simulink model "TV_lisb"  (R2024b)
settings: Solver=ode45  StartTime=0.0  StopTime=10  MaxStep=0.05  RelTol=1e-3
model workspace: external: MATLAB File C:\Users\USER\Documents\MATLAB\NR\TV_lisb_helper_file.m (data not in the file)
values from neighbouring files (symbols this model uses):
  b = 0.1    [TV_lisb_helper_file.m]
  C1 = 1.28    [TV_lisb_helper_file.m]
  C2 = 23.99    [TV_lisb_helper_file.m]
  C3 = 0.52    [TV_lisb_helper_file.m]
  C_d = 0.89    [TV_lisb_helper_file.m]
  C_roll = 0.01    [TV_lisb_helper_file.m]
  frontal_area = 1.35    [TV_lisb_helper_file.m]
  g = 9.8    [TV_lisb_helper_file.m]
  I_w = 1.5    [TV_lisb_helper_file.m]
  Izz = 3000    [TV_lisb_helper_file.m]
  lf = 1.5    [TV_lisb_helper_file.m]
  lr = 1.5    [TV_lisb_helper_file.m]
  M = 300    [TV_lisb_helper_file.m]
  rho = 1.223    [TV_lisb_helper_file.m]
  tr = 1    [TV_lisb_helper_file.m]
  wr = 0.22    [TV_lisb_helper_file.m]
libraries: simulink x1
(part 1 of 2)
settings Model: SnapshotBufferSize=100  SnapshotInterval=1  Creator=USER  LastModifiedBy=USER

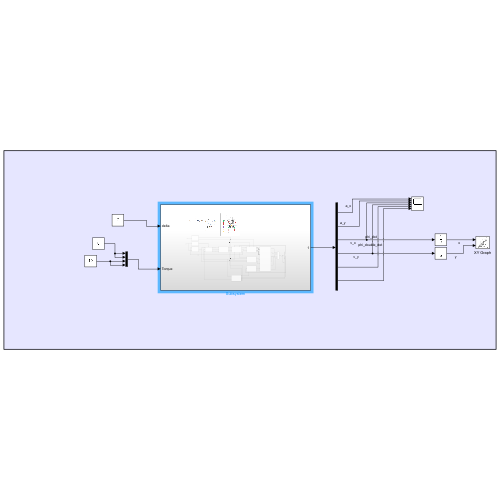
[thumbnail: Simulink's stored preview of the top-level diagram]
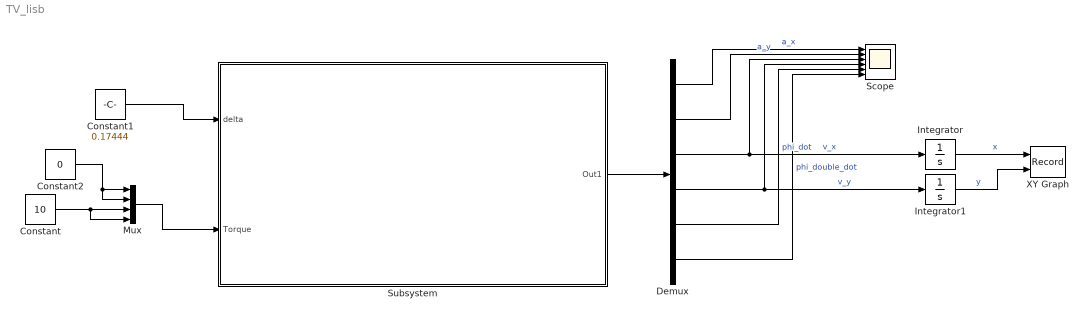
== system TV_lisb ==
  Constant : Constant  Value=10
  Constant1 : Constant  Value=0.17444
  Constant2 : Constant  Value=0
  Demux : Demux  Outputs=6
  Integrator : Integrator
  Integrator1 : Integrator
  Mux : Mux
  Scope : Scope  NumInputPorts=6
  Subsystem : Subsystem
  XY Graph : Record  FileSettingsInternal="{\"entries\":[{\"content\":{\"excelSettings\":{\"content\":{},\"type\":\"Streamout.ExcelSettings\"}},\"type\":\"Streamout.FileSettingStorage\",\"uuid\":\"\"}],\"packageUris\":[\"http:\\/\\/schema.mathworks.com\\/mf0\\/streamout_blocks\\/R2020a\"],\"version\":\"1.0\"}"  Layout=[1 1]  SignalsInternal="{\"entries\":[{\"content\":{\"signals\":[{\"content\":{\"blockPath\":[],\"dimensions\":[1],\"domain\":\"\",\"lineColor\":\"#a2142f\",\"plots\":[ 1 ],\"port\":1,\"sid\":[\"\"],\"signalID\":1,\"signalName\":\"x\"},\"type\":\"RecordBlkView.Signal\",\"uuid\":\"\"},{\"content\":{\"blockPath\":[],\"dimensions\":[1],\"domain\":\"\",\"lineColor\":\"#139fff\",\"plots\":[ 1 ],\"port\":2,\"sid\":[\"\"],\"signalID\":2,\"signalName\":\"y\"},\"type\":\"RecordBlkView.Signal\",\"uuid\":\"\"}]},\"type\":\"RecordBlkView.InputSignals\",\"uuid\":\"\"}],\"packageUris\":[\"http:\\/\\/schema.mathworks.com\\/mf0\\/streamout_blocks\\/R2020a\"],\"version\":\"1.0\"}"  VisualizationBindings="{\"xyplotplugin\":{\"info\":[{\"series\":[{\"bindingParametersList\":[{\"parameter\":\"X-Axis\",\"signalID\":1,\"signalName\":\"x\"},{\"parameter\":\"Y-Axis\",\"signalID\":2,\"signalName\":\"y\"}],\"seriesID\":0}],\"subplotID\":1}]}}"  CompatibilityTag=XY
  wires:
  Subsystem/1(Out1) -> Demux/1
  Demux/1 -> Scope/1  "a_x"
  Demux/2 -> Scope/2  "a_y"
  Demux/3 -> Scope/3, Integrator/1  "v_x"
  Demux/4 -> Scope/4, Integrator1/1  "v_y"
  Demux/5 -> Scope/5  "phi_dot"
  Demux/6 -> Scope/6  "phi_double_dot"
  Integrator/1 -> XY Graph/1  "x"
  Integrator1/1 -> XY Graph/2  "y"
  Constant1/1 -> Subsystem/1(delta)
  Mux/1 -> Subsystem/2(Torque)
  Constant/1 -> Mux/4, Mux/3
  Constant2/1 -> Mux/1, Mux/2

== system TV_lisb/Subsystem ==
  delta : Inport
  Torque : Inport  Port=2
  Accelerating_or_braking : Subsystem
  Aerodynamic Drag : Subsystem
  Demux : Demux  Outputs=6
  Mux : Mux  Inputs=6
      settings: DisplayOption=signals
  Rolling resistance : Subsystem
  Side Slip Angle : Subsystem
  Slip Ratios : Subsystem
      settings: PortSchema="{\"entries\":[{\"content\":{\"sides\":[{\"content\":{\"connectorIds\":[\"In1\",\"In2\",\"In3\"]},\"type\":\"ConnectorPlacement.EquallySpacedRectSide\",\"uuid\":\"f68f1183-9c60-479b-925c-3d4ffcaa1183\"},{\"content\":{\"connectorIds\":[\"Out1\",\"Out2\",\"Out3\"],\"side\":\"RIGHT\"},\"type\":\"ConnectorPlacement.EquallySpacedRectSide\",\"uuid\":\"3ccc78e5-55f6-4f64-bd15-35f9b9c5843d\"},{\"content\":{\"connectorIds\":[\"In4\"],\"side\":\"TOP\"},\"type\":\"ConnectorPlacement.EquallySpacedRectSide\",\"uuid\":\"873faff7-faeb-472b-bbf0-059c7e3a1cec\"}]},\"type\":\"ConnectorPlacement.EquallySpacedConnector\",\"uuid\":\"c1430164-14ee-465b-ad5a-b929bb7f1d2a\"}],\"packageUris\":[\"http://schema.mathworks.com/mf0/Connector/R2020b\"],\"version\":\"1.0\"}"
  Steering Kinematics : Subsystem
  Tire Model : Subsystem
  Torque and force equilibrium : Subsystem
  Unit Delay : UnitDelay  SampleTime=-1  HasFrameUpgradeWarning=on
  Unit Delay2 : UnitDelay  SampleTime=-1  HasFrameUpgradeWarning=on
  Vertical Loads : Subsystem
      settings: PortSchema="{\"entries\":[{\"content\":{\"sides\":[{\"content\":{\"connectorIds\":[\"In1\",\"In2\"]},\"type\":\"ConnectorPlacement.EquallySpacedRectSide\",\"uuid\":\"420474dd-77ae-41a3-b184-b8a376845dee\"},{\"content\":{\"connectorIds\":[\"Out1\",\"Out2\",\"Out3\"],\"side\":\"RIGHT\"},\"type\":\"ConnectorPlacement.EquallySpacedRectSide\",\"uuid\":\"e98bfd49-6816-4384-b726-feedfd108428\"},{\"content\":{\"connectorIds\":[\"In3\",\"In4\"],\"side\":\"TOP\"},\"type\":\"ConnectorPlacement.EquallySpacedRectSide\",\"uuid\":\"bc3c4692-54cb-49d4-bb5f-a504cda1efb8\"},{\"content\":{\"connectorIds\":[\"In5\",\"Out4\"],\"side\":\"BOTTOM\"},\"type\":\"ConnectorPlacement.EquallySpacedRectSide\",\"uuid\":\"ec39efe8-9589-4d25-8c83-c5c7b2f70cfd\"}]},\"type\":\"ConnectorPlacement.EquallySpacedConnector\",\"uuid\":\"6b01247e-c69a-46fe-b6d9-037bfd45934f\"}],\"packageUris\":[\"http://schema.mathworks.com/mf0/Connector/R2020b\"],\"version\":\"1.0\"}"
  Wheel Dynamics : Subsystem
  Wheel To Vehicle Co-ordinate System : Subsystem
      settings: PortSchema="{\"entries\":[{\"content\":{\"sides\":[{\"content\":{\"connectorIds\":[\"In1\",\"In2\"]},\"type\":\"ConnectorPlacement.EquallySpacedRectSide\",\"uuid\":\"1d639fc9-362c-4114-a9a5-2cccb0aa4f8f\"},{\"content\":{\"connectorIds\":[\"Out1\",\"Out2\"],\"side\":\"RIGHT\"},\"type\":\"ConnectorPlacement.EquallySpacedRectSide\",\"uuid\":\"af7b8bc1-4639-4e57-ae25-0425d451201b\"},{\"content\":{\"connectorIds\":[\"In3\",\"In4\"],\"side\":\"TOP\"},\"type\":\"ConnectorPlacement.EquallySpacedRectSide\",\"uuid\":\"e7928f69-bff2-45cc-8c36-948ca369821c\"}]},\"type\":\"ConnectorPlacement.EquallySpacedConnector\",\"uuid\":\"c77d5f9f-6196-466d-893b-8bb143925d68\"}],\"packageUris\":[\"http://schema.mathworks.com/mf0/Connector/R2020b\"],\"version\":\"1.0\"}"
  Out1 : Outport
  wires:
  Steering Kinematics/1(delta_left) -> Side Slip Angle/4(delta_l), Rolling resistance/2(delta_left), Wheel To Vehicle Co-ordinate System/4(delta_left)
  Vertical Loads/4(Total_z_force) -> Rolling resistance/1(Total_z_force)
  Steering Kinematics/2(delta_right) -> Side Slip Angle/5(delta_r), Rolling resistance/3(delta_right), Wheel To Vehicle Co-ordinate System/3(delta_right)
  Accelerating_or_braking/1(Binary state) -> Slip Ratios/4(Binary state)
  Torque and force equilibrium/4(v_y) -> Mux/4  "v_y"
  Side Slip Angle/1(alpha) -> Slip Ratios/2(Alpha), Vertical Loads/5(alpha)
  Slip Ratios/3(Slip_ratio_lateral) -> Tire Model/3(Slip_ratio_lateral)
  Wheel To Vehicle Co-ordinate System/2(Wheel_forces_y_wrt_body) -> Torque and force equilibrium/2(Wheel_forces_y_wrt_body)
  Rolling resistance/1(Rolling_force_x_body) -> Torque and force equilibrium/3(Rolling_force_x_body)
  Torque and force equilibrium/3(v_x) -> Mux/3  "v_x"
  Aerodynamic Drag/1(F_body_drag) -> Torque and force equilibrium/5(F_body_drag)
  Tire Model/1(mu_longitudinal) -> Vertical Loads/1(mu_longitudinal)
  Wheel To Vehicle Co-ordinate System/1(Wheel_forces_x_wrt_body) -> Torque and force equilibrium/1(Wheel_forces_x_wrt_body)
  Slip Ratios/1(Slip_ratio_resultant) -> Tire Model/1(Slip_ratio_resultant)
  Vertical Loads/3(Wheel_force_res) -> Unit Delay2/1
  Torque and force equilibrium/5(phi_dot) -> Mux/5  "phi_dot"
  Tire Model/2(mu_lateral) -> Vertical Loads/2(mu_lateral)
  Torque and force equilibrium/6(phi_double_dot) -> Mux/6  "phi_double_dot"
  Side Slip Angle/2(Wheel_velocity) -> Slip Ratios/3(Wheel velocity)
  Rolling resistance/2(Rolling_force_y_body) -> Torque and force equilibrium/4(Rolling_force_y_body)
  Slip Ratios/2(Slip_ratio_longitudinal) -> Tire Model/2(Slip_ratio_longitudinal)
  Vertical Loads/2(Wheel_force_y) -> Wheel To Vehicle Co-ordinate System/2(Wheel_force_y)
  Vertical Loads/1(Wheel_force_x) -> Wheel To Vehicle Co-ordinate System/1(Wheel_force_x)
  delta/1 -> Steering Kinematics/1(delta)
  Torque and force equilibrium/1(a_x) -> Mux/1  "a_x"
  Torque and force equilibrium/2(a_y) -> Mux/2  "a_y"
  Demux/2 -> Vertical Loads/3(Acceleration_y)
  Demux/1 -> Vertical Loads/4(Acceleration_x)
  Mux/1 -> Unit Delay/1
  Unit Delay/1 -> Out1/1, Demux/1
  Wheel Dynamics/1(omega) -> Slip Ratios/1(Omega), Rolling resistance/4(omega)
  Unit Delay2/1 -> Wheel Dynamics/1(Wheel_forces)
  Demux/3 -> Side Slip Angle/1(v_x), Aerodynamic Drag/1(v_x)
  Demux/4 -> Side Slip Angle/2(v_y)
  Demux/5 -> Side Slip Angle/3(phi_dot)
  Torque/1 -> Wheel Dynamics/2(Torque), Accelerating_or_braking/1(Torque)

== system TV_lisb/Subsystem/Accelerating_or_braking ==
  Torque : Inport
  Add : Sum
  Compare To Zero : simulink/Logic and Bit Operations/Compare To Zero  relop=>=  OutDataTypeStr=uint8
  Demux : Demux
  Derivative : Derivative
  Gain : Gain  Gain=0.5
  Binary state : Outport
  wires:
  Add/1 -> Gain/1
  Gain/1 -> Derivative/1
  Derivative/1 -> Compare To Zero/1
  Compare To Zero/1 -> Binary state/1
  Torque/1 -> Demux/1
  Demux/3 -> Add/1
  Demux/4 -> Add/2

== system TV_lisb/Subsystem/Aerodynamic Drag ==
  note: Aero calcs
  v_x : Inport
  Constant : Constant  Value=C_d
  Constant1 : Constant  Value=rho
  Gain : Gain  Gain=0.5
  Product : Product  Inputs=4
  Square : Math  Operator=square
  frontal area : Constant  Value=frontal_area
  F_body_drag : Outport
  wires:
  v_x/1 -> Square/1
  Product/1 -> Gain/1
  Square/1 -> Product/1
  Constant/1 -> Product/4
  Gain/1 -> F_body_drag/1
  Constant1/1 -> Product/3
  frontal area/1 -> Product/2

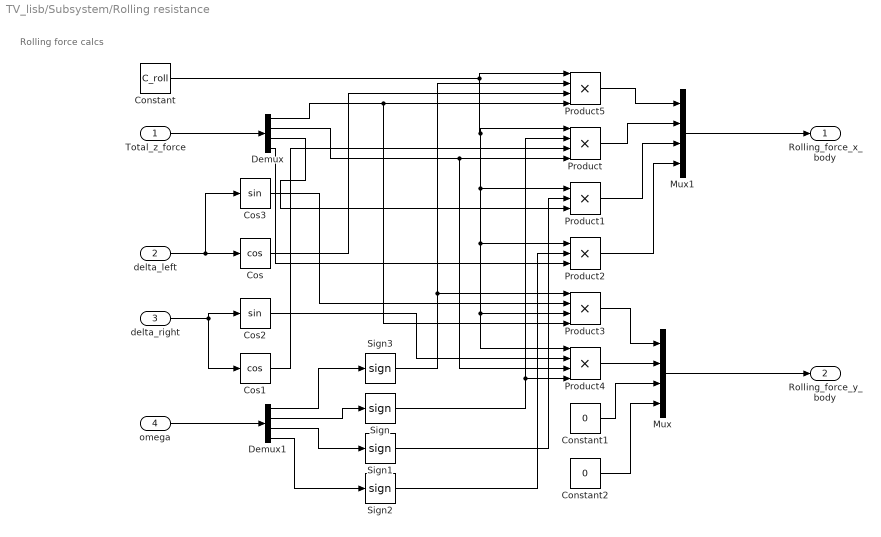
== system TV_lisb/Subsystem/Rolling resistance ==
  note: Rolling force calcs
  Total_z_force : Inport
  delta_left : Inport  Port=2
  delta_right : Inport  Port=3
  omega : Inport  Port=4
  Constant : Constant  Value=C_roll
  Constant1 : Constant  Value=0
  Constant2 : Constant  Value=0
  Cos : Trigonometry  Operator=cos
  Cos1 : Trigonometry  Operator=cos
  Cos2 : Trigonometry
  Cos3 : Trigonometry
  Demux : Demux
  Demux1 : Demux
  Mux : Mux
  Mux1 : Mux
  Product{,3..5} (4 alike) : Product  Inputs=4
  Product1 : Product  Inputs=3
  Product2 : Product  Inputs=3
  Sign{,1..3} (4 alike) : Signum
  Rolling_force_x_body : Outport
  Rolling_force_y_body : Outport  Port=2
  wires:
  Total_z_force/1 -> Demux/1
  omega/1 -> Demux1/1
  delta_left/1 -> Cos3/1, Cos/1
  delta_right/1 -> Cos2/1, Cos1/1
  Demux1/1 -> Sign3/1
  Demux1/2 -> Sign/1
  Demux1/3 -> Sign1/1
  Demux1/4 -> Sign2/1
  Constant/1 -> Product4/1, Product3/3, Product2/1, Product1/1, Product/1, Product5/1
  Demux/1 -> Product3/4, Product5/4
  Sign3/1 -> Product3/1, Product5/2
  Cos/1 -> Product5/3
  Demux/2 -> Product4/3, Product/4
  Sign/1 -> Product/2, Product4/4
  Cos1/1 -> Product/3
  Demux/3 -> Product1/3
  Demux/4 -> Product2/3
  Sign1/1 -> Product1/2
  Sign2/1 -> Product2/2
  Mux1/1 -> Rolling_force_x_body/1
  Product5/1 -> Mux1/1
  Product/1 -> Mux1/2
  Product1/1 -> Mux1/3
  Product2/1 -> Mux1/4
  Mux/1 -> Rolling_force_y_body/1
  Constant2/1 -> Mux/4
  Constant1/1 -> Mux/3
  Product4/1 -> Mux/2
  Product3/1 -> Mux/1
  Cos3/1 -> Product3/2
  Cos2/1 -> Product4/2

== system TV_lisb/Subsystem/Side Slip Angle ==
  note: Slip angle calcs
  v_x : Inport
  v_y : Inport  Port=2
  phi_dot : Inport  Port=3
  delta_l : Inport  Port=4
  delta_r : Inport  Port=5
  Constant : Constant  Value=lr
  Constant1 : Constant  Value=lf
  Constant2 : Constant  Value=tf
  Constant3 : Constant  Value=tr
  R_calcs : Subsystem
  alpha1 : Subsystem
      settings: PortSchema="{\"entries\":[{\"content\":{\"sides\":[{\"content\":{\"connectorIds\":[\"In1\",\"In2\",\"In3\",\"In4\",\"In5\"]},\"type\":\"ConnectorPlacement.EquallySpacedRectSide\",\"uuid\":\"8658fdab-e6e4-4ff2-af71-2cb52fa4d16f\"},{\"content\":{\"connectorIds\":[\"Out1\"],\"side\":\"RIGHT\"},\"type\":\"ConnectorPlacement.EquallySpacedRectSide\",\"uuid\":\"0155b14f-1735-45fb-b67c-bf6dca8000dd\"},{\"content\":{\"side\":\"TOP\"},\"type\":\"ConnectorPlacement.EquallySpacedRectSide\",\"uuid\":\"ae187582-448a-4e1f-8e59-a94c37e4b1d5\"},{\"content\":{\"connectorIds\":[\"In6\",\"In7\"],\"side\":\"BOTTOM\"},\"type\":\"ConnectorPlacement.EquallySpacedRectSide\",\"uuid\":\"ea241970-7db7-4bad-a15f-ddecb92249c5\"}]},\"type\":\"ConnectorPlacement.EquallySpacedConnector\",\"uuid\":\"3ec76c52-149c-4fb2-a8d0-51517714a4be\"}],\"packageUris\":[\"http://schema.mathworks.com/mf0/Connector/R2020b\"],\"version\":\"1.0\"}"
  eta_calcs : Subsystem
  w_v : Subsystem
  alpha : Outport
  Wheel_velocity : Outport  Port=2
  wires:
  Constant2/1 -> R_calcs/1(tf), eta_calcs/1(tf)
  Constant1/1 -> eta_calcs/2(lf), R_calcs/2(lf)
  Constant/1 -> R_calcs/3(lr), eta_calcs/3(lr)
  Constant3/1 -> R_calcs/4(tr), eta_calcs/4(tr)
  w_v/1(wheel_velocity) -> Wheel_velocity/1
  alpha1/1(alpha) -> alpha/1
  eta_calcs/1(eta) -> w_v/1(eta), alpha1/1(eta)
  R_calcs/1(R) -> w_v/2(R), alpha1/2(R)
  v_x/1 -> alpha1/3(v_x), w_v/3(v_x)
  v_y/1 -> alpha1/4(v_y), w_v/4(v_y)
  phi_dot/1 -> alpha1/5(phi_dot), w_v/5(phi_dot)
  delta_l/1 -> alpha1/6(delta_l)
  delta_r/1 -> alpha1/7(delta_r)

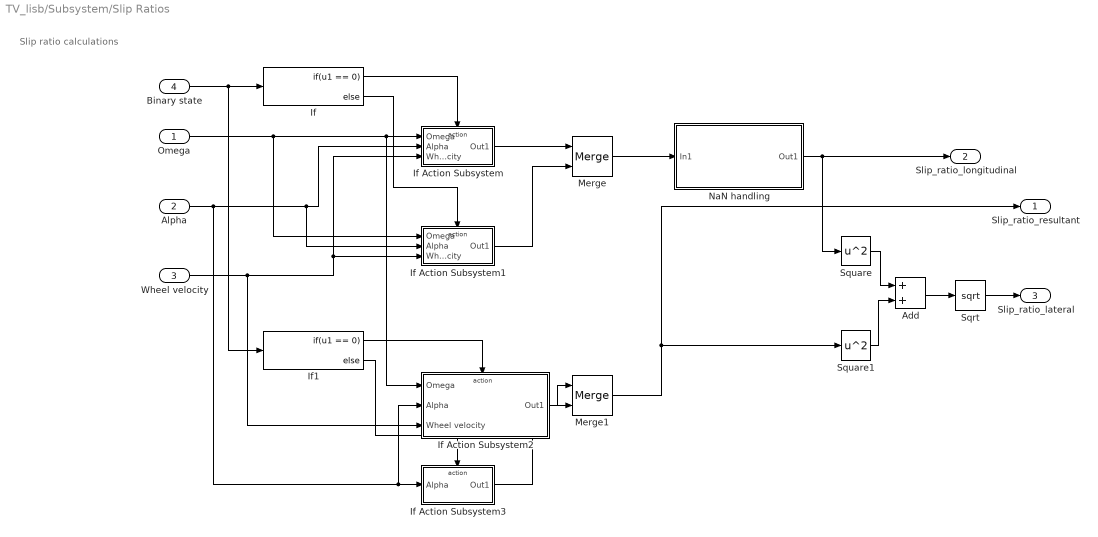
== system TV_lisb/Subsystem/Slip Ratios ==
  note: Slip ratio calculations
  Omega : Inport
  Alpha : Inport  Port=2
  Wheel velocity : Inport  Port=3
  Binary state : Inport  Port=4
  Add : Sum
  If : If  IfExpression=u1 == 0
  If Action Subsystem : Subsystem  TreatAsAtomicUnit=on
  If Action Subsystem1 : Subsystem  TreatAsAtomicUnit=on
  If Action Subsystem2 : Subsystem  TreatAsAtomicUnit=on
  If Action Subsystem3 : Subsystem  TreatAsAtomicUnit=on
  If1 : If  IfExpression=u1 == 0
  Merge : Merge
  Merge1 : Merge
  NaN handling : Subsystem
  Sqrt : Sqrt
  Square : Math  Operator=square
  Square1 : Math  Operator=square
  Slip_ratio_resultant : Outport
  Slip_ratio_longitudinal : Outport  Port=2
  Slip_ratio_lateral : Outport  Port=3
  wires:
  Binary state/1 -> If/1, If1/1
  If/1 -> If Action Subsystem/Action
  If/2 -> If Action Subsystem1/Action
  Omega/1 -> If Action Subsystem2/1(Omega), If Action Subsystem/1(Omega), If Action Subsystem1/1(Omega)
  Alpha/1 -> If Action Subsystem1/2(Alpha), If Action Subsystem/2(Alpha), If Action Subsystem2/2(Alpha), If Action Subsystem3/1(Alpha)
  Wheel velocity/1 -> If Action Subsystem2/3(Wheel velocity), If Action Subsystem1/3(Wheel velocity), If Action Subsystem/3(Wheel velocity)
  If Action Subsystem/1(Out1) -> Merge/1
  If Action Subsystem1/1(Out1) -> Merge/2
  Merge/1 -> NaN handling/1(In1)
  If Action Subsystem2/1(Out1) -> Merge1/1
  If Action Subsystem3/1(Out1) -> Merge1/2
  Merge1/1 -> Slip_ratio_resultant/1, Square1/1
  If1/1 -> If Action Subsystem2/Action
  If1/2 -> If Action Subsystem3/Action
  Sqrt/1 -> Slip_ratio_lateral/1
  Add/1 -> Sqrt/1
  Square/1 -> Add/1
  Square1/1 -> Add/2
  NaN handling/1(Out1) -> Square/1, Slip_ratio_longitudinal/1

== system TV_lisb/Subsystem/Steering Kinematics ==
  delta : Inport
  If : If  IfExpression=u1 ~= 0
  If Action Subsystem : Subsystem  TreatAsAtomicUnit=on
  If Action Subsystem1 : Subsystem  TreatAsAtomicUnit=on
  Merge : Merge
  Merge1 : Merge
  delta_left : Outport
  delta_right : Outport  Port=2
  wires:
  delta/1 -> If Action Subsystem/1(delta), If/1
  If/1 -> If Action Subsystem/Action
  If Action Subsystem/1(delta_l) -> Merge/1
  Merge/1 -> delta_left/1
  If Action Subsystem/2(delta_r) -> Merge1/1
  Merge1/1 -> delta_right/1
  If/2 -> If Action Subsystem1/Action
  If Action Subsystem1/2(Out2) -> Merge1/2
  If Action Subsystem1/1(Out1) -> Merge/2

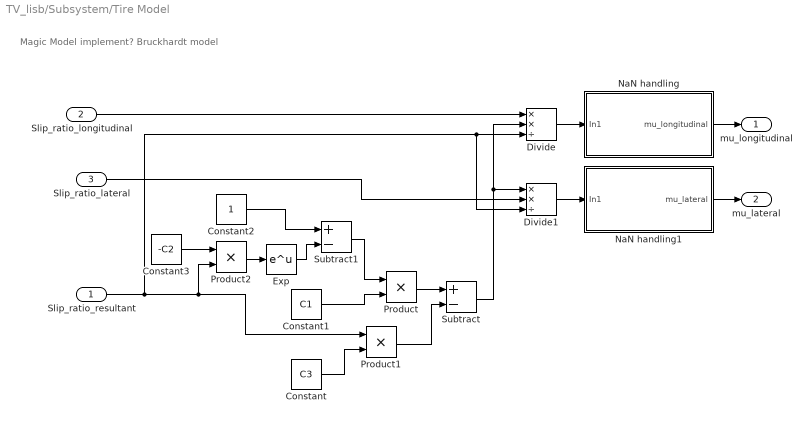
== system TV_lisb/Subsystem/Tire Model ==
  note: Magic Model implement?
      | Bruckhardt model
  Slip_ratio_resultant : Inport
  Slip_ratio_longitudinal : Inport  Port=2
  Slip_ratio_lateral : Inport  Port=3
  Constant : Constant  Value=C3
  Constant1 : Constant  Value=C1
  Constant2 : Constant
  Constant3 : Constant  Value=-C2
  Divide : Product  Inputs=**/
  Divide1 : Product  Inputs=**/
  Exp : Math
  NaN handling : Subsystem
  NaN handling1 : Subsystem
  Product : Product
  Product1 : Product
  Product2 : Product
  Subtract : Sum  Inputs=+-
  Subtract1 : Sum  Inputs=+-
  mu_longitudinal : Outport
  mu_lateral : Outport  Port=2
  wires:
  Product/1 -> Subtract/1
  Product1/1 -> Subtract/2
  Subtract/1 -> Divide1/1, Divide/2
  Slip_ratio_resultant/1 -> Divide1/3, Divide/3, Product2/2, Product1/1
  Constant/1 -> Product1/2
  Constant1/1 -> Product/2
  Subtract1/1 -> Product/1
  Constant2/1 -> Subtract1/1
  Constant3/1 -> Product2/1
  Exp/1 -> Subtract1/2
  Product2/1 -> Exp/1
  Slip_ratio_longitudinal/1 -> Divide/1
  Slip_ratio_lateral/1 -> Divide1/2
  NaN handling1/1(mu_lateral) -> mu_lateral/1
  Divide1/1 -> NaN handling1/1(In1)
  Divide/1 -> NaN handling/1(In1)
  NaN handling/1(mu_longitudinal) -> mu_longitudinal/1

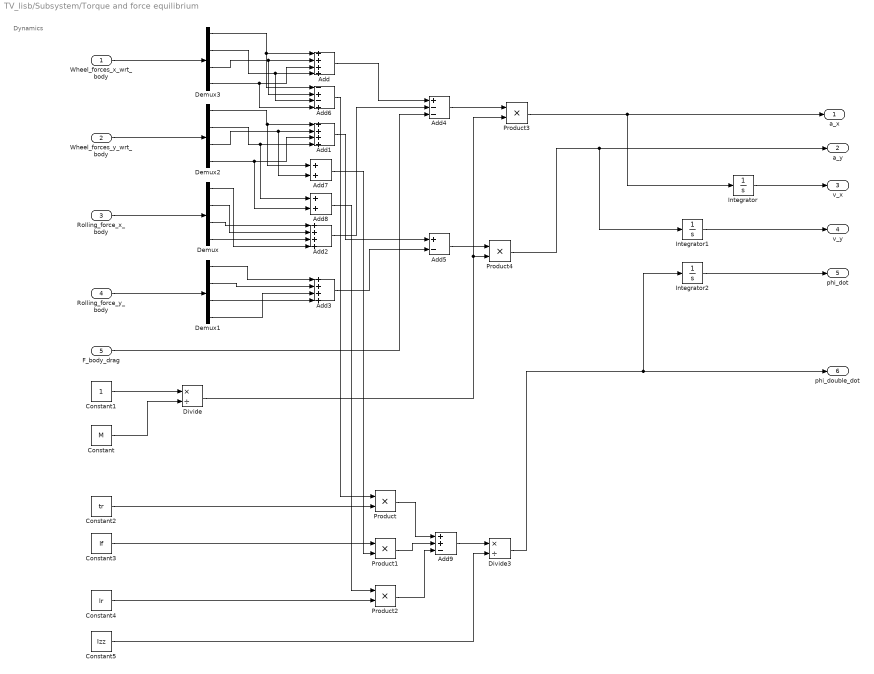
== system TV_lisb/Subsystem/Torque and force equilibrium ==
  note: Dynamics
  Wheel_forces_x_wrt_body : Inport
  Wheel_forces_y_wrt_body : Inport  Port=2
  Rolling_force_x_body : Inport  Port=3
  Rolling_force_y_body : Inport  Port=4
  F_body_drag : Inport  Port=5
  Add{,1..3} (4 alike) : Sum  Inputs=++++
  Add4 : Sum  Inputs=+--
  Add5 : Sum  Inputs=+-
  Add6 : Sum  Inputs=-+-+
  Add7 : Sum
  Add8 : Sum
  Add9 : Sum  Inputs=++-
  Constant : Constant  Value=M
  Constant1 : Constant
  Constant2 : Constant  Value=tr
  Constant3 : Constant  Value=lf
  Constant4 : Constant  Value=lr
  Constant5 : Constant  Value=Izz
  Demux{,1..3} (4 alike) : Demux
  Divide : Product  Inputs=*/
  Divide3 : Product  Inputs=*/
  Integrator : Integrator
  Integrator1 : Integrator
  Integrator2 : Integrator
  Product{,1..4} (5 alike) : Product
  a_x : Outport
  a_y : Outport  Port=2
  v_x : Outport  Port=3
  v_y : Outport  Port=4
  phi_dot : Outport  Port=5
  phi_double_dot : Outport  Port=6
  wires:
  Wheel_forces_x_wrt_body/1 -> Demux3/1
  Wheel_forces_y_wrt_body/1 -> Demux2/1
  Rolling_force_x_body/1 -> Demux/1
  Rolling_force_y_body/1 -> Demux1/1
  Demux3/1 -> Add6/1, Add/1
  Demux3/2 -> Add6/3, Add/4
  Demux3/3 -> Add6/2, Add/2
  Demux3/4 -> Add6/4, Add/3
  Demux2/1 -> Add7/1, Add1/1
  Demux2/2 -> Add8/1, Add1/4
  Demux2/3 -> Add7/2, Add1/2
  Demux2/4 -> Add8/2, Add1/3
  Demux/1 -> Add2/4
  Demux/2 -> Add2/2
  Demux/3 -> Add2/1
  Demux/4 -> Add2/3
  Demux1/1 -> Add3/1
  Demux1/2 -> Add3/2
  Demux1/3 -> Add3/4
  Demux1/4 -> Add3/3
  Add/1 -> Add4/1
  Add2/1 -> Add4/2
  F_body_drag/1 -> Add4/3
  Add1/1 -> Add5/1
  Add3/1 -> Add5/2
  Constant1/1 -> Divide/1
  Constant/1 -> Divide/2
  Divide/1 -> Product4/2, Product3/2
  Add4/1 -> Product3/1
  Add5/1 -> Product4/1
  Product3/1 -> Integrator/1, a_x/1
  Product4/1 -> Integrator1/1, a_y/1
  Integrator/1 -> v_x/1
  Integrator1/1 -> v_y/1
  Divide3/1 -> phi_double_dot/1, Integrator2/1
  Integrator2/1 -> phi_dot/1
  Add6/1 -> Product/1
  Constant2/1 -> Product/2
  Product/1 -> Add9/1
  Product1/1 -> Add9/2
  Product2/1 -> Add9/3
  Add9/1 -> Divide3/1
  Constant5/1 -> Divide3/2
  Constant3/1 -> Product1/1
  Constant4/1 -> Product2/2
  Add7/1 -> Product1/2
  Add8/1 -> Product2/1

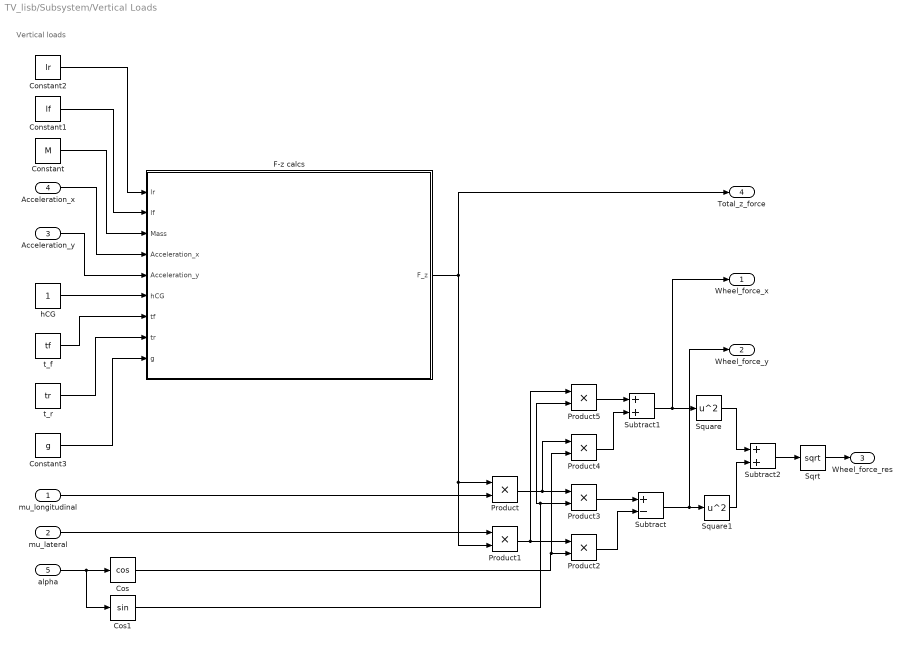
== system TV_lisb/Subsystem/Vertical Loads ==
  note: Vertical loads
  mu_longitudinal : Inport
  mu_lateral : Inport  Port=2
  Acceleration_y : Inport  Port=3
  Acceleration_x : Inport  Port=4
  alpha : Inport  Port=5
  Constant : Constant  Value=M
  Constant1 : Constant  Value=lf
  Constant2 : Constant  Value=lr
  Constant3 : Constant  Value=g
  Cos : Trigonometry  Operator=cos
  Cos1 : Trigonometry
  F-z calcs : Subsystem
  Product{,1..5} (6 alike) : Product
  Sqrt : Sqrt
  Square : Math  Operator=square
  Square1 : Math  Operator=square
  Subtract : Sum  Inputs=+-
  Subtract1 : Sum
  Subtract2 : Sum
  hCG : Constant
  t_f : Constant  Value=tf
  t_r : Constant  Value=tr
  Wheel_force_x : Outport
  Wheel_force_y : Outport  Port=2
  Wheel_force_res : Outport  Port=3
  Total_z_force : Outport  Port=4
  wires:
  Constant/1 -> F-z calcs/3(Mass)
  Constant2/1 -> F-z calcs/1(lr)
  Constant1/1 -> F-z calcs/2(lf)
  Acceleration_x/1 -> F-z calcs/4(Acceleration_x)
  Acceleration_y/1 -> F-z calcs/5(Acceleration_y)
  hCG/1 -> F-z calcs/6(hCG)
  t_f/1 -> F-z calcs/7(tf)
  Constant3/1 -> F-z calcs/9(g)
  t_r/1 -> F-z calcs/8(tr)
  F-z calcs/1(F_z) -> Product1/2, Product/1, Total_z_force/1
  mu_longitudinal/1 -> Product/2
  mu_lateral/1 -> Product1/1
  alpha/1 -> Cos1/1, Cos/1
  Cos/1 -> Product4/2, Product2/2
  Product1/1 -> Product5/1, Product2/1
  Product/1 -> Product4/1, Product3/1
  Cos1/1 -> Product5/2, Product3/2
  Product3/1 -> Subtract/1
  Product2/1 -> Subtract/2
  Subtract/1 -> Square1/1, Wheel_force_y/1
  Product5/1 -> Subtract1/1
  Product4/1 -> Subtract1/2
  Subtract1/1 -> Square/1, Wheel_force_x/1
  Subtract2/1 -> Sqrt/1
  Square1/1 -> Subtract2/2
  Square/1 -> Subtract2/1
  Sqrt/1 -> Wheel_force_res/1

== system TV_lisb/Subsystem/Wheel Dynamics ==
  Wheel_forces : Inport
  Torque : Inport  Port=2
  Add : Sum  Inputs=+--
  Constant1 : Constant  Value=wr
  Constant2 : Constant  Value=b
  Constant3 : Constant  Value=I_w
  Divide : Product  Inputs=*/
  Integrator : Integrator
  Product : Product
  Product1 : Product
  omega : Outport
  wires:
  Integrator/1 -> Product1/2, omega/1
  Torque/1 -> Add/1
  Wheel_forces/1 -> Product/1
  Constant1/1 -> Product/2
  Product/1 -> Add/2
  Constant2/1 -> Product1/1
  Product1/1 -> Add/3
  Add/1 -> Divide/1
  Divide/1 -> Integrator/1
  Constant3/1 -> Divide/2

== system TV_lisb/Subsystem/Wheel To Vehicle Co-ordinate System ==
  note: Co-ordinate calculations
  Wheel_force_x : Inport
  Wheel_force_y : Inport  Port=2
  delta_right : Inport  Port=3
  delta_left : Inport  Port=4
  Subsystem : Subsystem
  Subsystem1 : Subsystem
  Wheel_forces_x_wrt_body : Outport
  Wheel_forces_y_wrt_body : Outport  Port=2
  wires:
  Wheel_force_x/1 -> Subsystem1/1(Wheel_force_x), Subsystem/1(Wheel_force_x)
  delta_right/1 -> Subsystem1/3(delta_right), Subsystem/3(delta_right)
  delta_left/1 -> Subsystem1/4(delta_left), Subsystem/4(delta_left)
  Wheel_force_y/1 -> Subsystem/2(Wheel_force_y), Subsystem1/2(Wheel_force_y)
  Subsystem/1(Wheel_forces_x_wrt_body) -> Wheel_forces_x_wrt_body/1
  Subsystem1/1(Wheel_forces_y_wrt_body) -> Wheel_forces_y_wrt_body/1

== system TV_lisb/Subsystem/Side Slip Angle/R_calcs ==
  tf : Inport
  lf : Inport  Port=2
  lr : Inport  Port=3
  tr : Inport  Port=4
  Add : Sum
  Add1 : Sum
  Mux : Mux  Inputs=2
  Sqrt : Sqrt
  Sqrt1 : Sqrt
  Square{,1..3} (4 alike) : Math  Operator=square
  R : Outport
  wires:
  Add/1 -> Sqrt/1
  Sqrt/1 -> Mux/1
  Square/1 -> Add/1
  Square1/1 -> Add/2
  Square2/1 -> Add1/1
  Sqrt1/1 -> Mux/2
  Square3/1 -> Add1/2
  Add1/1 -> Sqrt1/1
  tf/1 -> Square/1
  lf/1 -> Square1/1
  lr/1 -> Square2/1
  tr/1 -> Square3/1
  Mux/1 -> R/1

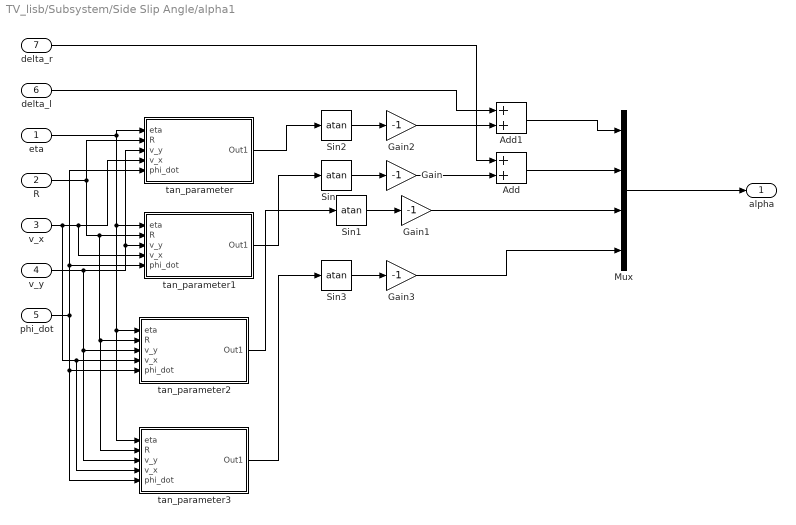
== system TV_lisb/Subsystem/Side Slip Angle/alpha1 ==
  eta : Inport
  R : Inport  Port=2
  v_x : Inport  Port=3
  v_y : Inport  Port=4
  phi_dot : Inport  Port=5
  delta_l : Inport  Port=6
  delta_r : Inport  Port=7
  Add : Sum
  Add1 : Sum
  Gain{,1..3} (4 alike) : Gain  Gain=-1
  Mux : Mux
  Sin{,1..3} (4 alike) : Trigonometry  Operator=atan
  tan_parameter : Subsystem
  tan_parameter1 : Subsystem
  tan_parameter2 : Subsystem
  tan_parameter3 : Subsystem
  alpha : Outport
  wires:
  Mux/1 -> alpha/1
  Sin/1 -> Gain/1
  Gain3/1 -> Mux/4
  Gain1/1 -> Mux/3
  Gain/1 -> Add/2
  Gain2/1 -> Add1/2
  Add/1 -> Mux/2
  Add1/1 -> Mux/1
  delta_l/1 -> Add1/1
  delta_r/1 -> Add/1
  Sin1/1 -> Gain1/1
  Sin3/1 -> Gain3/1
  Sin2/1 -> Gain2/1
  tan_parameter/1(Out1) -> Sin2/1
  tan_parameter1/1(Out1) -> Sin/1
  tan_parameter2/1(Out1) -> Sin1/1
  tan_parameter3/1(Out1) -> Sin3/1
  eta/1 -> tan_parameter3/1(eta), tan_parameter2/1(eta), tan_parameter1/1(eta), tan_parameter/1(eta)
  R/1 -> tan_parameter3/2(R), tan_parameter2/2(R), tan_parameter1/2(R), tan_parameter/2(R)
  v_x/1 -> tan_parameter3/4(v_x), tan_parameter2/4(v_x), tan_parameter1/4(v_x), tan_parameter/4(v_x)
  v_y/1 -> tan_parameter3/3(v_y), tan_parameter2/3(v_y), tan_parameter1/3(v_y), tan_parameter/3(v_y)
  phi_dot/1 -> tan_parameter3/5(phi_dot), tan_parameter2/5(phi_dot), tan_parameter1/5(phi_dot), tan_parameter/5(phi_dot)

== system TV_lisb/Subsystem/Side Slip Angle/eta_calcs ==
  tf : Inport
  lf : Inport  Port=2
  lr : Inport  Port=3
  tr : Inport  Port=4
  Divide{,1..3} (4 alike) : Product  Inputs=*/
  Mux : Mux
  Sin{,1..3} (4 alike) : Trigonometry  Operator=atan
  eta : Outport
  wires:
  Sin1/1 -> Mux/2
  Divide1/1 -> Sin1/1
  lf/1 -> Divide1/1, Divide/2
  tr/1 -> Divide3/1, Divide2/2
  Divide2/1 -> Sin2/1
  tf/1 -> Divide1/2, Divide/1
  Divide/1 -> Sin/1
  lr/1 -> Divide3/2, Divide2/1
  Divide3/1 -> Sin3/1
  Sin/1 -> Mux/1
  Sin3/1 -> Mux/4
  Sin2/1 -> Mux/3
  Mux/1 -> eta/1

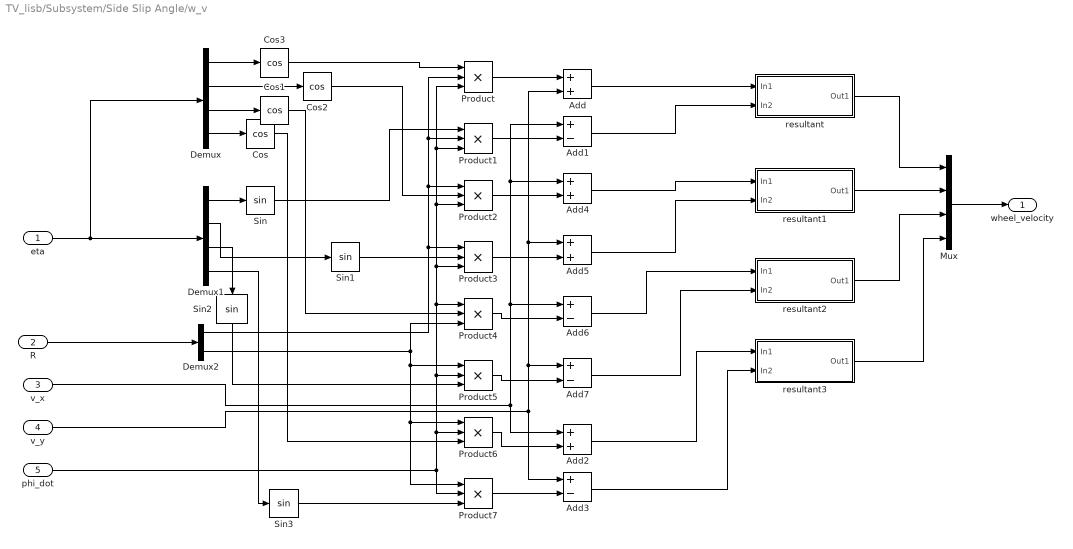
== system TV_lisb/Subsystem/Side Slip Angle/w_v ==
  eta : Inport
  R : Inport  Port=2
  v_x : Inport  Port=3
  v_y : Inport  Port=4
  phi_dot : Inport  Port=5
  Add{,2,4..5} (4 alike) : Sum
  Add{1,3,6..7} (4 alike) : Sum  Inputs=+-
  Cos{,1..3} (4 alike) : Trigonometry  Operator=cos
  Demux : Demux
  Demux1 : Demux
  Demux2 : Demux  Outputs=2
  Mux : Mux
  Product{,1..7} (8 alike) : Product  Inputs=3
  Sin{,1..3} (4 alike) : Trigonometry
  resultant : Subsystem
  resultant1 : Subsystem
  resultant2 : Subsystem
  resultant3 : Subsystem
  wheel_velocity : Outport
  wires:
  phi_dot/1 -> Product7/2, Product6/2, Product5/2, Product4/1, Product3/3, Product2/3, Product1/3, Product/3
  R/1 -> Demux2/1
  eta/1 -> Demux1/1, Demux/1
  resultant/1(Out1) -> Mux/1
  Mux/1 -> wheel_velocity/1
  resultant1/1(Out1) -> Mux/2
  resultant2/1(Out1) -> Mux/3
  resultant3/1(Out1) -> Mux/4
  Demux2/1 -> Product3/1, Product2/1, Product1/2, Product/2
  Demux/1 -> Cos3/1
  Demux1/1 -> Sin/1
  Product/1 -> Add/1
  v_y/1 -> Add3/1, Add7/1, Add5/1, Add/2
  Add/1 -> resultant/1(In1)
  Product1/1 -> Add1/2
  v_x/1 -> Add6/1, Add4/1, Add1/1, Add2/1
  Add1/1 -> resultant/2(In2)
  Demux2/2 -> Product5/1, Product6/1, Product7/1, Product4/3
  Product2/1 -> Add4/2
  Product3/1 -> Add5/2
  Product4/1 -> Add6/2
  Product5/1 -> Add7/2
  Product6/1 -> Add2/2
  Product7/1 -> Add3/2
  Add4/1 -> resultant1/1(In1)
  Add5/1 -> resultant1/2(In2)
  Add6/1 -> resultant2/1(In1)
  Add7/1 -> resultant2/2(In2)
  Add2/1 -> resultant3/1(In1)
  Add3/1 -> resultant3/2(In2)
  Demux/2 -> Cos2/1
  Demux1/2 -> Sin1/1
  Demux/3 -> Cos1/1
  Demux1/3 -> Sin2/1
  Demux/4 -> Cos/1
  Demux1/4 -> Sin3/1
  Cos/1 -> Product6/3
  Cos1/1 -> Product4/2
  Cos2/1 -> Product2/2
  Cos3/1 -> Product/1
  Sin/1 -> Product1/1
  Sin1/1 -> Product3/2
  Sin2/1 -> Product5/3
  Sin3/1 -> Product7/3

== system TV_lisb/Subsystem/Slip Ratios/If Action Subsystem ==
  Omega : Inport
  Alpha : Inport  Port=2
  Wheel velocity : Inport  Port=3
  Action Port : ActionPort  ActionPortLabel=if(u1 == 0)
  Constant : Constant  Value=wr
  Cos : Trigonometry  Operator=cos
  Divide : Product  Inputs=*/
  Product : Product  Inputs=3
  Subtract : Sum  Inputs=+-
  Out1 : Outport
  wires:
  Constant/1 -> Product/1
  Omega/1 -> Product/2
  Alpha/1 -> Cos/1
  Cos/1 -> Product/3
  Product/1 -> Subtract/1
  Wheel velocity/1 -> Divide/2, Subtract/2
  Subtract/1 -> Divide/1
  Divide/1 -> Out1/1

== system TV_lisb/Subsystem/Slip Ratios/If Action Subsystem1 ==
  Omega : Inport
  Alpha : Inport  Port=2
  Wheel velocity : Inport  Port=3
  Action Port : ActionPort  ActionPortLabel=else
  Constant : Constant  Value=wr
  Cos : Trigonometry  Operator=cos
  Divide : Product  Inputs=*/
  Product : Product  Inputs=3
  Subtract : Sum  Inputs=+-
  Out1 : Outport
  wires:
  Product/1 -> Divide/2, Subtract/1
  Subtract/1 -> Divide/1
  Alpha/1 -> Cos/1
  Cos/1 -> Product/3
  Omega/1 -> Product/2
  Constant/1 -> Product/1
  Divide/1 -> Out1/1
  Wheel velocity/1 -> Subtract/2

== system TV_lisb/Subsystem/Slip Ratios/If Action Subsystem2 ==
  Omega : Inport
  Alpha : Inport  Port=2
  Wheel velocity : Inport  Port=3
  Action Port : ActionPort  ActionPortLabel=if(u1 == 0)
  Constant : Constant  Value=wr
  Cos : Trigonometry
  Divide : Product  Inputs=*/
  Product : Product  Inputs=3
  Out1 : Outport
  wires:
  Constant/1 -> Product/1
  Omega/1 -> Product/2
  Alpha/1 -> Cos/1
  Cos/1 -> Product/3
  Wheel velocity/1 -> Divide/2
  Product/1 -> Divide/1
  Divide/1 -> Out1/1

== system TV_lisb/Subsystem/Slip Ratios/If Action Subsystem3 ==
  Alpha : Inport
  Action Port : ActionPort  ActionPortLabel=else
  Tan : Trigonometry  Operator=tan
  Out1 : Outport
  wires:
  Alpha/1 -> Tan/1
  Tan/1 -> Out1/1

== system TV_lisb/Subsystem/Slip Ratios/NaN handling ==
  In1 : Inport
  Demux : Demux
  Mux : Mux
  Subsystem : Subsystem
  Subsystem1 : Subsystem
  Subsystem2 : Subsystem
  Subsystem3 : Subsystem
  Out1 : Outport
  wires:
  In1/1 -> Demux/1
  Subsystem/1(Out1) -> Mux/1
  Subsystem1/1(Out1) -> Mux/2
  Subsystem2/1(Out1) -> Mux/3
  Subsystem3/1(Out1) -> Mux/4
  Mux/1 -> Out1/1
  Demux/1 -> Subsystem/1(In1)
  Demux/2 -> Subsystem1/1(In1)
  Demux/3 -> Subsystem2/1(In1)
  Demux/4 -> Subsystem3/1(In1)

== system TV_lisb/Subsystem/Steering Kinematics/If Action Subsystem ==
  delta : Inport
  Action Port : ActionPort  ActionPortLabel=if(u1 ~= 0)
  Add : Sum
  Add1 : Sum
  Add2 : Sum  Inputs=+-
  Constant : Constant
  Constant1 : Constant  Value=lf
  Constant2 : Constant  Value=lr
  Constant3 : Constant  Value=tf
  Divide : Product  Inputs=*/
  Divide1 : Product  Inputs=*/
  Divide2 : Product  Inputs=*/
  Gain : Gain  Gain=1/2
  Product : Product
  Tan : Trigonometry  Operator=atan
  Tan1 : Trigonometry  Operator=tan
  Tan2 : Trigonometry  Operator=atan
  delta_l : Outport
  delta_r : Outport  Port=2
  wires:
  Add1/1 -> Divide1/2
  Constant/1 -> Divide/1
  Add2/1 -> Divide2/2
  Divide/1 -> Product/1
  Constant2/1 -> Add/2
  Product/1 -> Add2/1, Add1/1
  Gain/1 -> Add2/2, Add1/2
  Tan1/1 -> Divide/2
  Divide2/1 -> Tan2/1
  delta/1 -> Tan1/1
  Divide1/1 -> Tan/1
  Tan/1 -> delta_l/1
  Constant1/1 -> Add/1
  Constant3/1 -> Gain/1
  Add/1 -> Divide1/1, Divide2/1, Product/2
  Tan2/1 -> delta_r/1

== system TV_lisb/Subsystem/Steering Kinematics/If Action Subsystem1 ==
  Action Port : ActionPort  ActionPortLabel=else
  Constant : Constant  Value=0
  Signal Copy : SignalConversion  OverrideOpt=off
  Signal Copy1 : SignalConversion  OverrideOpt=off
  Out1 : Outport
  Out2 : Outport  Port=2
  wires:
  Signal Copy1/1 -> Out2/1
  Signal Copy/1 -> Out1/1
  Constant/1 -> Signal Copy1/1, Signal Copy/1

== system TV_lisb/Subsystem/Tire Model/NaN handling ==
  In1 : Inport
  Demux : Demux
  Mux : Mux
  Subsystem : Subsystem
  Subsystem1 : Subsystem
  Subsystem2 : Subsystem
  Subsystem3 : Subsystem
  mu_longitudinal : Outport
  wires:
  In1/1 -> Demux/1
  Mux/1 -> mu_longitudinal/1
  Demux/1 -> Subsystem/1(In1)
  Demux/2 -> Subsystem1/1(In1)
  Demux/3 -> Subsystem2/1(In1)
  Demux/4 -> Subsystem3/1(In1)
  Subsystem/1(Out1) -> Mux/1
  Subsystem1/1(Out1) -> Mux/2
  Subsystem2/1(Out1) -> Mux/3
  Subsystem3/1(Out1) -> Mux/4

== system TV_lisb/Subsystem/Tire Model/NaN handling1 ==
  In1 : Inport
  Demux : Demux
  Mux : Mux
  Subsystem : Subsystem
  Subsystem1 : Subsystem
  Subsystem2 : Subsystem
  Subsystem3 : Subsystem
  mu_lateral : Outport
  wires:
  In1/1 -> Demux/1
  Mux/1 -> mu_lateral/1
  Demux/1 -> Subsystem/1(In1)
  Demux/2 -> Subsystem1/1(In1)
  Demux/3 -> Subsystem2/1(In1)
  Demux/4 -> Subsystem3/1(In1)
  Subsystem/1(Out1) -> Mux/1
  Subsystem1/1(Out1) -> Mux/2
  Subsystem2/1(Out1) -> Mux/3
  Subsystem3/1(Out1) -> Mux/4

== system TV_lisb/Subsystem/Vertical Loads/F-z calcs ==
  lr : Inport
  lf : Inport  Port=2
  Mass : Inport  Port=3
  Acceleration_x : Inport  Port=4
  Acceleration_y : Inport  Port=5
  hCG : Inport  Port=6
  tf : Inport  Port=7
  tr : Inport  Port=8
  g : Inport  Port=9
  Mux : Mux
  Product{,1..3} (4 alike) : Product  Inputs=3
  Term_1 : Subsystem
  Term_2 : Subsystem
  F_z : Outport
  wires:
  lr/1 -> Term_1/1(lr)
  Acceleration_x/1 -> Term_1/2(Acceleration_x)
  lf/1 -> Term_1/3(lf)
  hCG/1 -> Term_2/1(hCG), Term_1/4(hCG)
  g/1 -> Term_2/2(g), Term_1/5(g)
  Acceleration_y/1 -> Term_2/5(Acceleration_y)
  tf/1 -> Term_2/4(tf)
  tr/1 -> Term_2/3(tr)
  Product/1 -> Mux/1
  Product1/1 -> Mux/2
  Product2/1 -> Mux/3
  Product3/1 -> Mux/4
  Mass/1 -> Product3/1, Product2/1, Product1/1, Product/1
  Term_1/2(minus) -> Product1/2, Product/3
  Term_2/2(minus_f) -> Product/2
  Term_2/1(plus_f) -> Product1/3
  Term_1/1(plus) -> Product3/2, Product2/2
  Term_2/4(minus_r) -> Product2/3
  Term_2/3(plus_r) -> Product3/3
  Mux/1 -> F_z/1

== system TV_lisb/Subsystem/Wheel To Vehicle Co-ordinate System/Subsystem ==
  Wheel_force_x : Inport
  Wheel_force_y : Inport  Port=2
  delta_right : Inport  Port=3
  delta_left : Inport  Port=4
  Bus Creator : BusCreator  Inputs=4
  Cos : Trigonometry  Operator=cos
  Cos1 : Trigonometry
  Cos2 : Trigonometry  Operator=cos
  Cos3 : Trigonometry
  Demux : Demux
  Demux1 : Demux
  Product{,1..3} (4 alike) : Product
  Subtract : Sum  Inputs=+-
  Subtract1 : Sum  Inputs=+-
  Wheel_forces_x_wrt_body : Outport
  wires:
  Demux/1 -> Product/2
  Demux/3 -> Bus Creator/3
  Wheel_force_x/1 -> Demux/1
  Demux/4 -> Bus Creator/4
  Bus Creator/1 -> Wheel_forces_x_wrt_body/1
  delta_left/1 -> Cos/1, Cos1/1
  Cos/1 -> Product/1
  Product/1 -> Subtract/1
  Cos1/1 -> Product1/2
  Wheel_force_y/1 -> Demux1/1
  Demux1/1 -> Product1/1
  Product1/1 -> Subtract/2
  Subtract/1 -> Bus Creator/1
  delta_right/1 -> Cos3/1, Cos2/1
  Product2/1 -> Subtract1/1
  Product3/1 -> Subtract1/2
  Subtract1/1 -> Bus Creator/2
  Demux/2 -> Product2/1
  Cos2/1 -> Product2/2
  Demux1/2 -> Product3/1
  Cos3/1 -> Product3/2

== system TV_lisb/Subsystem/Wheel To Vehicle Co-ordinate System/Subsystem1 ==
  Wheel_force_x : Inport
  Wheel_force_y : Inport  Port=2
  delta_right : Inport  Port=3
  delta_left : Inport  Port=4
  Add : Sum
  Add1 : Sum
  Bus Creator : BusCreator  Inputs=4
  Demux : Demux
  Demux1 : Demux
  Product{,1..3} (4 alike) : Product
  Sin : Trigonometry  Operator=cos
  Sin1 : Trigonometry
  Sin2 : Trigonometry
  Sin3 : Trigonometry  Operator=cos
  Wheel_forces_y_wrt_body : Outport
  wires:
  Demux1/2 -> Product2/1
  Demux1/1 -> Product/1
  Demux1/3 -> Bus Creator/3
  Wheel_force_y/1 -> Demux1/1
  Demux1/4 -> Bus Creator/4
  Bus Creator/1 -> Wheel_forces_y_wrt_body/1
  Wheel_force_x/1 -> Demux/1
  delta_right/1 -> Sin/1, Sin1/1
  delta_left/1 -> Sin3/1, Sin2/1
  Product2/1 -> Add1/1
  Product3/1 -> Add1/2
  Product/1 -> Add/1
  Product1/1 -> Add/2
  Add/1 -> Bus Creator/1
  Add1/1 -> Bus Creator/2
  Sin3/1 -> Product/2
  Demux/1 -> Product1/1
  Sin2/1 -> Product1/2
  Sin/1 -> Product2/2
  Demux/2 -> Product3/1
  Sin1/1 -> Product3/2

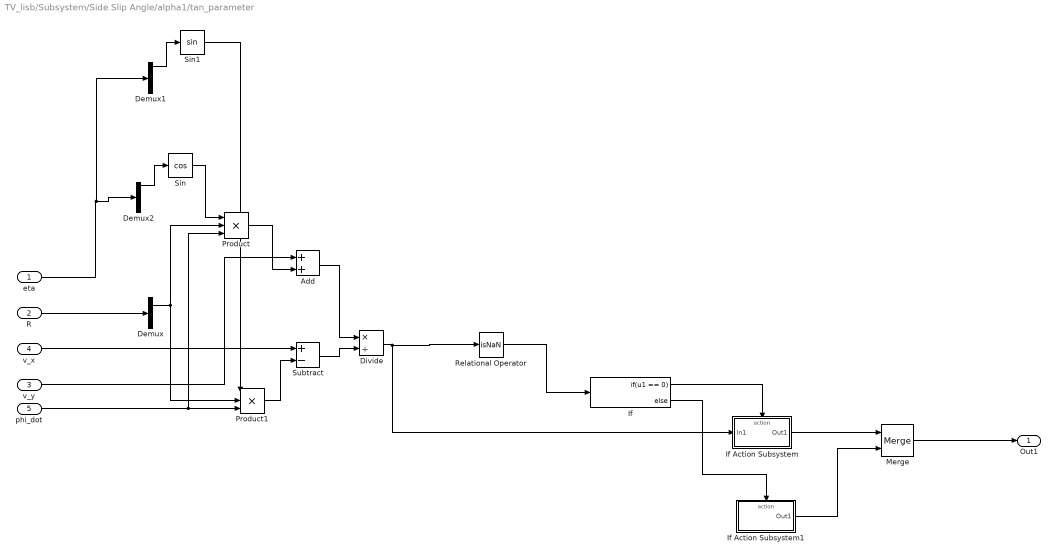
== system TV_lisb/Subsystem/Side Slip Angle/alpha1/tan_parameter ==
  eta : Inport
  R : Inport  Port=2
  v_y : Inport  Port=3
  v_x : Inport  Port=4
  phi_dot : Inport  Port=5
  Add : Sum
  Demux : Demux  Outputs=2
  Demux1 : Demux
  Demux2 : Demux
  Divide : Product  Inputs=*/
  If : If  IfExpression=u1 == 0
  If Action Subsystem : Subsystem  TreatAsAtomicUnit=on
  If Action Subsystem1 : Subsystem  TreatAsAtomicUnit=on
  Merge : Merge
  Product : Product  Inputs=3
  Product1 : Product  Inputs=3
  Relational Operator : RelationalOperator  Operator=isNaN  OutDataTypeStr=boolean  RndMeth=Simplest  InputSameDT=off
  Sin : Trigonometry  Operator=cos
  Sin1 : Trigonometry
  Subtract : Sum  Inputs=+-
  Out1 : Outport
  wires:
  R/1 -> Demux/1
  eta/1 -> Demux2/1, Demux1/1
  Divide/1 -> Relational Operator/1, If Action Subsystem/1(In1)
  Add/1 -> Divide/1
  Subtract/1 -> Divide/2
  v_y/1 -> Add/1
  Product/1 -> Add/2
  v_x/1 -> Subtract/1
  Product1/1 -> Subtract/2
  phi_dot/1 -> Product/3, Product1/3
  Demux/1 -> Product1/2, Product/2
  Demux2/1 -> Sin/1
  Demux1/1 -> Sin1/1
  Sin1/1 -> Product1/1
  Sin/1 -> Product/1
  If/1 -> If Action Subsystem/Action
  If/2 -> If Action Subsystem1/Action
  If Action Subsystem/1(Out1) -> Merge/1
  If Action Subsystem1/1(Out1) -> Merge/2
  Merge/1 -> Out1/1
  Relational Operator/1 -> If/1

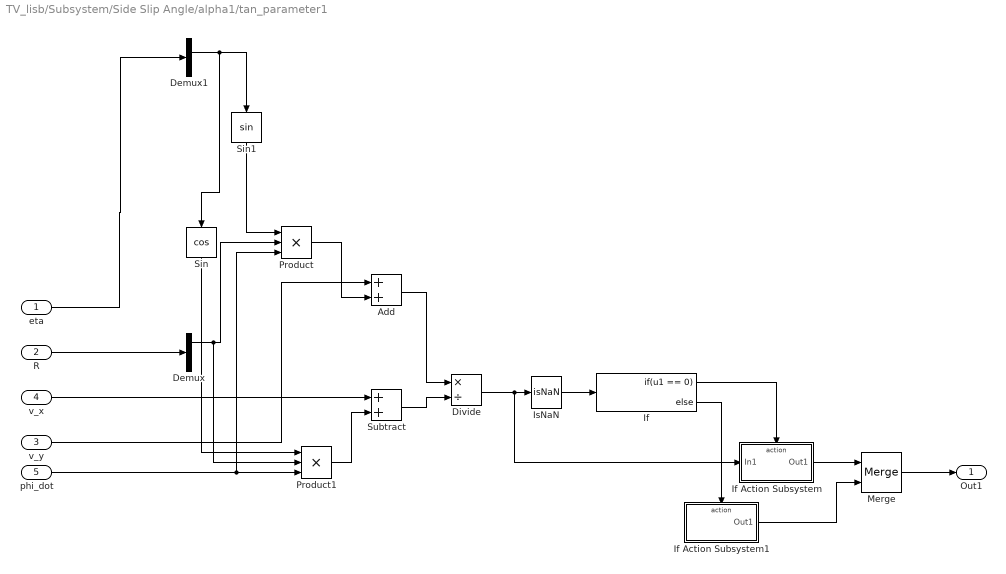
== system TV_lisb/Subsystem/Side Slip Angle/alpha1/tan_parameter1 ==
  eta : Inport
  R : Inport  Port=2
  v_y : Inport  Port=3
  v_x : Inport  Port=4
  phi_dot : Inport  Port=5
  Add : Sum
  Demux : Demux  Outputs=2
  Demux1 : Demux
  Divide : Product  Inputs=*/
  If : If  IfExpression=u1 == 0
  If Action Subsystem : Subsystem  TreatAsAtomicUnit=on
  If Action Subsystem1 : Subsystem  TreatAsAtomicUnit=on
  IsNaN : RelationalOperator  Operator=isNaN  OutDataTypeStr=boolean  RndMeth=Simplest  InputSameDT=off
  Merge : Merge
  Product : Product  Inputs=3
  Product1 : Product  Inputs=3
  Sin : Trigonometry  Operator=cos
  Sin1 : Trigonometry
  Subtract : Sum
  Out1 : Outport
  wires:
  R/1 -> Demux/1
  eta/1 -> Demux1/1
  Add/1 -> Divide/1
  Subtract/1 -> Divide/2
  v_y/1 -> Add/1
  Product/1 -> Add/2
  v_x/1 -> Subtract/1
  Product1/1 -> Subtract/2
  phi_dot/1 -> Product/3, Product1/3
  Demux/1 -> Product1/2, Product/2
  Demux1/2 -> Sin/1, Sin1/1
  Sin/1 -> Product1/1
  Sin1/1 -> Product/1
  Divide/1 -> If Action Subsystem/1(In1), IsNaN/1
  IsNaN/1 -> If/1
  If/1 -> If Action Subsystem/Action
  If/2 -> If Action Subsystem1/Action
  If Action Subsystem/1(Out1) -> Merge/1
  If Action Subsystem1/1(Out1) -> Merge/2
  Merge/1 -> Out1/1

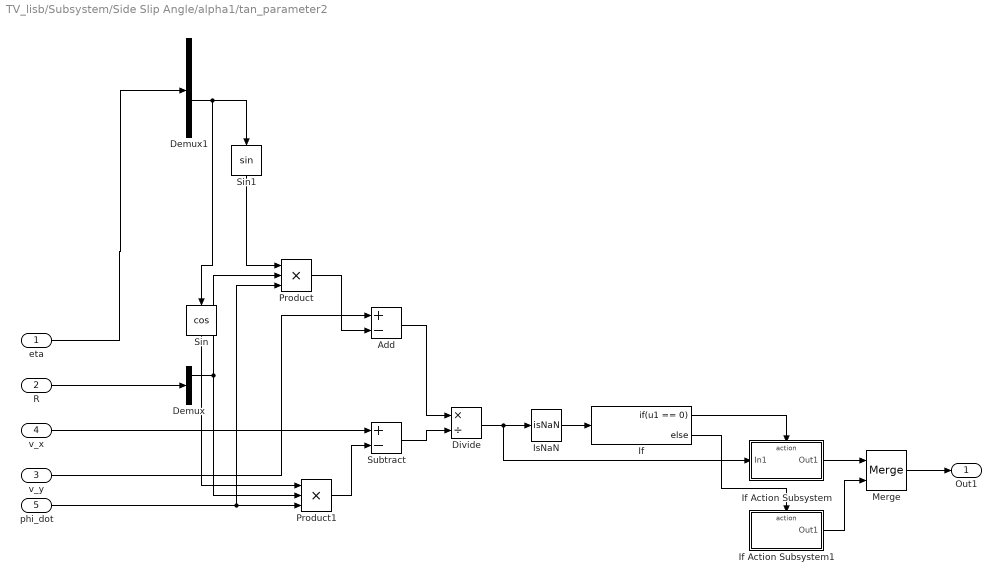
== system TV_lisb/Subsystem/Side Slip Angle/alpha1/tan_parameter2 ==
  eta : Inport
  R : Inport  Port=2
  v_y : Inport  Port=3
  v_x : Inport  Port=4
  phi_dot : Inport  Port=5
  Add : Sum  Inputs=+-
  Demux : Demux  Outputs=2
  Demux1 : Demux
  Divide : Product  Inputs=*/
  If : If  IfExpression=u1 == 0
  If Action Subsystem : Subsystem  TreatAsAtomicUnit=on
  If Action Subsystem1 : Subsystem  TreatAsAtomicUnit=on
  IsNaN : RelationalOperator  Operator=isNaN  OutDataTypeStr=boolean  RndMeth=Simplest  InputSameDT=off
  Merge : Merge
  Product : Product  Inputs=3
  Product1 : Product  Inputs=3
  Sin : Trigonometry  Operator=cos
  Sin1 : Trigonometry
  Subtract : Sum  Inputs=+-
  Out1 : Outport
  wires:
  R/1 -> Demux/1
  eta/1 -> Demux1/1
  Divide/1 -> If Action Subsystem/1(In1), IsNaN/1
  Add/1 -> Divide/1
  Subtract/1 -> Divide/2
  v_y/1 -> Add/1
  Product/1 -> Add/2
  v_x/1 -> Subtract/1
  Product1/1 -> Subtract/2
  phi_dot/1 -> Product/3, Product1/3
  Demux/1 -> Product1/2, Product/2
  Demux1/3 -> Sin/1, Sin1/1
  Sin/1 -> Product1/1
  Sin1/1 -> Product/1
  IsNaN/1 -> If/1
  If/1 -> If Action Subsystem/Action
  If/2 -> If Action Subsystem1/Action
  If Action Subsystem/1(Out1) -> Merge/1
  If Action Subsystem1/1(Out1) -> Merge/2
  Merge/1 -> Out1/1

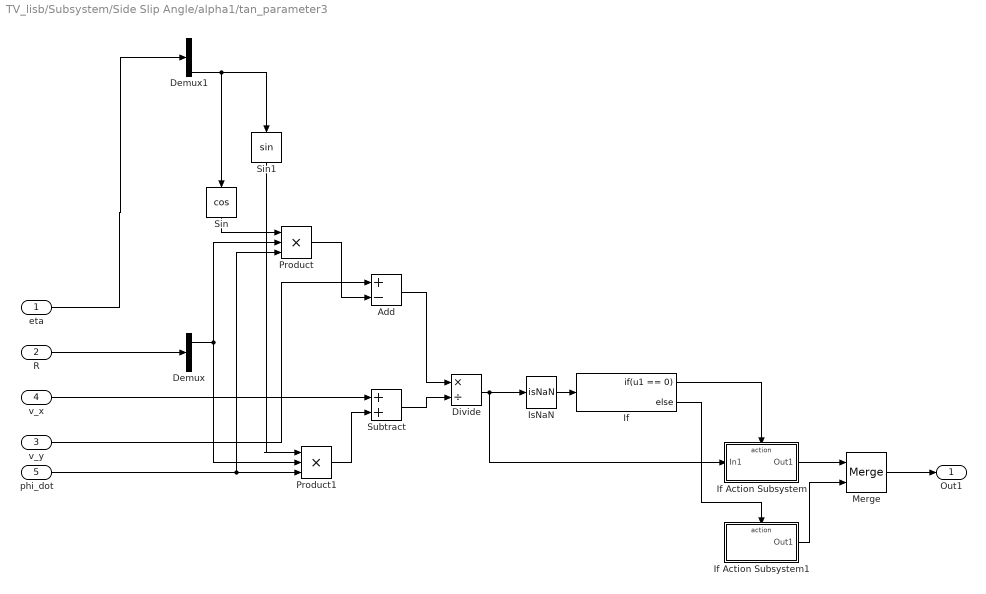
== system TV_lisb/Subsystem/Side Slip Angle/alpha1/tan_parameter3 ==
  eta : Inport
  R : Inport  Port=2
  v_y : Inport  Port=3
  v_x : Inport  Port=4
  phi_dot : Inport  Port=5
  Add : Sum  Inputs=+-
  Demux : Demux  Outputs=2
  Demux1 : Demux
  Divide : Product  Inputs=*/
  If : If  IfExpression=u1 == 0
  If Action Subsystem : Subsystem  TreatAsAtomicUnit=on
  If Action Subsystem1 : Subsystem  TreatAsAtomicUnit=on
  IsNaN : RelationalOperator  Operator=isNaN  OutDataTypeStr=boolean  RndMeth=Simplest  InputSameDT=off
  Merge : Merge
  Product : Product  Inputs=3
  Product1 : Product  Inputs=3
  Sin : Trigonometry  Operator=cos
  Sin1 : Trigonometry
  Subtract : Sum
  Out1 : Outport
  wires:
  R/1 -> Demux/1
  eta/1 -> Demux1/1
  Divide/1 -> If Action Subsystem/1(In1), IsNaN/1
  Add/1 -> Divide/1
  Subtract/1 -> Divide/2
  v_y/1 -> Add/1
  Product/1 -> Add/2
  v_x/1 -> Subtract/1
  Product1/1 -> Subtract/2
  phi_dot/1 -> Product/3, Product1/3
  Demux/1 -> Product1/2, Product/2
  Demux1/4 -> Sin1/1, Sin/1
  Sin/1 -> Product/1
  Sin1/1 -> Product1/1
  IsNaN/1 -> If/1
  If Action Subsystem/1(Out1) -> Merge/1
  If Action Subsystem1/1(Out1) -> Merge/2
  Merge/1 -> Out1/1
  If/1 -> If Action Subsystem/Action
  If/2 -> If Action Subsystem1/Action

== system TV_lisb/Subsystem/Side Slip Angle/w_v/resultant ==
  In1 : Inport
  In2 : Inport  Port=2
  Add : Sum
  Sqrt : Sqrt
  Square : Math  Operator=square
  Square1 : Math  Operator=square
  Out1 : Outport
  wires:
  In2/1 -> Square/1
  In1/1 -> Square1/1
  Square1/1 -> Add/1
  Square/1 -> Add/2
  Add/1 -> Sqrt/1
  Sqrt/1 -> Out1/1

== system TV_lisb/Subsystem/Side Slip Angle/w_v/resultant1 ==
  In1 : Inport
  In2 : Inport  Port=2
  Add : Sum
  Sqrt : Sqrt
  Square : Math  Operator=square
  Square1 : Math  Operator=square
  Out1 : Outport
  wires:
  In2/1 -> Square/1
  In1/1 -> Square1/1
  Square1/1 -> Add/1
  Square/1 -> Add/2
  Add/1 -> Sqrt/1
  Sqrt/1 -> Out1/1

== system TV_lisb/Subsystem/Side Slip Angle/w_v/resultant2 ==
  In1 : Inport
  In2 : Inport  Port=2
  Add : Sum
  Sqrt : Sqrt
  Square : Math  Operator=square
  Square1 : Math  Operator=square
  Out1 : Outport
  wires:
  In2/1 -> Square/1
  In1/1 -> Square1/1
  Square1/1 -> Add/1
  Square/1 -> Add/2
  Add/1 -> Sqrt/1
  Sqrt/1 -> Out1/1

== system TV_lisb/Subsystem/Side Slip Angle/w_v/resultant3 ==
  In1 : Inport
  In2 : Inport  Port=2
  Add : Sum
  Sqrt : Sqrt
  Square : Math  Operator=square
  Square1 : Math  Operator=square
  Out1 : Outport
  wires:
  In2/1 -> Square/1
  In1/1 -> Square1/1
  Square1/1 -> Add/1
  Square/1 -> Add/2
  Add/1 -> Sqrt/1
  Sqrt/1 -> Out1/1

== system TV_lisb/Subsystem/Slip Ratios/NaN handling/Subsystem ==
  In1 : Inport
  If : If  IfExpression=u1 == 0
  If Action Subsystem : Subsystem  TreatAsAtomicUnit=on
  If Action Subsystem1 : Subsystem  TreatAsAtomicUnit=on
  Merge : Merge
  Relational Operator : RelationalOperator  Operator=isNaN  OutDataTypeStr=boolean  RndMeth=Simplest  InputSameDT=off
  Out1 : Outport
  wires:
  If Action Subsystem1/1(Out1) -> Merge/2
  In1/1 -> If Action Subsystem/1(In1), Relational Operator/1
  Merge/1 -> Out1/1
  If/2 -> If Action Subsystem1/Action
  If/1 -> If Action Subsystem/Action
  If Action Subsystem/1(Out1) -> Merge/1
  Relational Operator/1 -> If/1

== system TV_lisb/Subsystem/Slip Ratios/NaN handling/Subsystem1 ==
  In1 : Inport
  If : If  IfExpression=u1 == 0
  If Action Subsystem : Subsystem  TreatAsAtomicUnit=on
  If Action Subsystem1 : Subsystem  TreatAsAtomicUnit=on
  Merge : Merge
  Relational Operator : RelationalOperator  Operator=isNaN  OutDataTypeStr=boolean  RndMeth=Simplest  InputSameDT=off
  Out1 : Outport
  wires:
  If Action Subsystem1/1(Out1) -> Merge/2
  In1/1 -> If Action Subsystem/1(In1), Relational Operator/1
  Merge/1 -> Out1/1
  If/2 -> If Action Subsystem1/Action
  If/1 -> If Action Subsystem/Action
  If Action Subsystem/1(Out1) -> Merge/1
  Relational Operator/1 -> If/1

== system TV_lisb/Subsystem/Slip Ratios/NaN handling/Subsystem2 ==
  In1 : Inport
  If : If  IfExpression=u1 == 0
  If Action Subsystem : Subsystem  TreatAsAtomicUnit=on
  If Action Subsystem1 : Subsystem  TreatAsAtomicUnit=on
  Merge : Merge
  Relational Operator : RelationalOperator  Operator=isNaN  OutDataTypeStr=boolean  RndMeth=Simplest  InputSameDT=off
  Out1 : Outport
  wires:
  If Action Subsystem1/1(Out1) -> Merge/2
  In1/1 -> If Action Subsystem/1(In1), Relational Operator/1
  Merge/1 -> Out1/1
  If/2 -> If Action Subsystem1/Action
  If/1 -> If Action Subsystem/Action
  If Action Subsystem/1(Out1) -> Merge/1
  Relational Operator/1 -> If/1

== system TV_lisb/Subsystem/Slip Ratios/NaN handling/Subsystem3 ==
  In1 : Inport
  If : If  IfExpression=u1 == 0
  If Action Subsystem : Subsystem  TreatAsAtomicUnit=on
  If Action Subsystem1 : Subsystem  TreatAsAtomicUnit=on
  Merge : Merge
  Relational Operator : RelationalOperator  Operator=isNaN  OutDataTypeStr=boolean  RndMeth=Simplest  InputSameDT=off
  Out1 : Outport
  wires:
  If Action Subsystem1/1(Out1) -> Merge/2
  In1/1 -> If Action Subsystem/1(In1), Relational Operator/1
  Merge/1 -> Out1/1
  If/2 -> If Action Subsystem1/Action
  If/1 -> If Action Subsystem/Action
  If Action Subsystem/1(Out1) -> Merge/1
  Relational Operator/1 -> If/1

== system TV_lisb/Subsystem/Tire Model/NaN handling/Subsystem ==
  In1 : Inport
  If : If  IfExpression=u1 == 0
  If Action Subsystem : Subsystem  TreatAsAtomicUnit=on
  If Action Subsystem1 : Subsystem  TreatAsAtomicUnit=on
  Merge : Merge
  Relational Operator : RelationalOperator  Operator=isNaN  OutDataTypeStr=boolean  RndMeth=Simplest  InputSameDT=off
  Out1 : Outport
  wires:
  If Action Subsystem1/1(Out1) -> Merge/2
  In1/1 -> If Action Subsystem/1(In1), Relational Operator/1
  Merge/1 -> Out1/1
  If/2 -> If Action Subsystem1/Action
  If/1 -> If Action Subsystem/Action
  If Action Subsystem/1(Out1) -> Merge/1
  Relational Operator/1 -> If/1

== system TV_lisb/Subsystem/Tire Model/NaN handling/Subsystem1 ==
  In1 : Inport
  If : If  IfExpression=u1 == 0
  If Action Subsystem : Subsystem  TreatAsAtomicUnit=on
  If Action Subsystem1 : Subsystem  TreatAsAtomicUnit=on
  Merge : Merge
  Relational Operator : RelationalOperator  Operator=isNaN  OutDataTypeStr=boolean  RndMeth=Simplest  InputSameDT=off
  Out1 : Outport
  wires:
  If Action Subsystem1/1(Out1) -> Merge/2
  In1/1 -> If Action Subsystem/1(In1), Relational Operator/1
  Merge/1 -> Out1/1
  If/2 -> If Action Subsystem1/Action
  If/1 -> If Action Subsystem/Action
  If Action Subsystem/1(Out1) -> Merge/1
  Relational Operator/1 -> If/1

== system TV_lisb/Subsystem/Tire Model/NaN handling/Subsystem2 ==
  In1 : Inport
  If : If  IfExpression=u1 == 0
  If Action Subsystem : Subsystem  TreatAsAtomicUnit=on
  If Action Subsystem1 : Subsystem  TreatAsAtomicUnit=on
  Merge : Merge
  Relational Operator : RelationalOperator  Operator=isNaN  OutDataTypeStr=boolean  RndMeth=Simplest  InputSameDT=off
  Out1 : Outport
  wires:
  If Action Subsystem1/1(Out1) -> Merge/2
  In1/1 -> If Action Subsystem/1(In1), Relational Operator/1
  Merge/1 -> Out1/1
  If/2 -> If Action Subsystem1/Action
  If/1 -> If Action Subsystem/Action
  If Action Subsystem/1(Out1) -> Merge/1
  Relational Operator/1 -> If/1

== system TV_lisb/Subsystem/Tire Model/NaN handling/Subsystem3 ==
  In1 : Inport
  If : If  IfExpression=u1 == 0
  If Action Subsystem : Subsystem  TreatAsAtomicUnit=on
  If Action Subsystem1 : Subsystem  TreatAsAtomicUnit=on
  Merge : Merge
  Relational Operator : RelationalOperator  Operator=isNaN  OutDataTypeStr=boolean  RndMeth=Simplest  InputSameDT=off
  Out1 : Outport
  wires:
  If Action Subsystem1/1(Out1) -> Merge/2
  In1/1 -> If Action Subsystem/1(In1), Relational Operator/1
  Merge/1 -> Out1/1
  If/2 -> If Action Subsystem1/Action
  If/1 -> If Action Subsystem/Action
  If Action Subsystem/1(Out1) -> Merge/1
  Relational Operator/1 -> If/1

== system TV_lisb/Subsystem/Tire Model/NaN handling1/Subsystem ==
  In1 : Inport
  If : If  IfExpression=u1 == 0
  If Action Subsystem : Subsystem  TreatAsAtomicUnit=on
  If Action Subsystem1 : Subsystem  TreatAsAtomicUnit=on
  Merge : Merge
  Relational Operator : RelationalOperator  Operator=isNaN  OutDataTypeStr=boolean  RndMeth=Simplest  InputSameDT=off
  Out1 : Outport
  wires:
  If Action Subsystem1/1(Out1) -> Merge/2
  In1/1 -> If Action Subsystem/1(In1), Relational Operator/1
  Merge/1 -> Out1/1
  If/2 -> If Action Subsystem1/Action
  If/1 -> If Action Subsystem/Action
  If Action Subsystem/1(Out1) -> Merge/1
  Relational Operator/1 -> If/1

== system TV_lisb/Subsystem/Tire Model/NaN handling1/Subsystem1 ==
  In1 : Inport
  If : If  IfExpression=u1 == 0
  If Action Subsystem : Subsystem  TreatAsAtomicUnit=on
  If Action Subsystem1 : Subsystem  TreatAsAtomicUnit=on
  Merge : Merge
  Relational Operator : RelationalOperator  Operator=isNaN  OutDataTypeStr=boolean  RndMeth=Simplest  InputSameDT=off
  Out1 : Outport
  wires:
  If Action Subsystem1/1(Out1) -> Merge/2
  In1/1 -> If Action Subsystem/1(In1), Relational Operator/1
  Merge/1 -> Out1/1
  If/2 -> If Action Subsystem1/Action
  If/1 -> If Action Subsystem/Action
  If Action Subsystem/1(Out1) -> Merge/1
  Relational Operator/1 -> If/1

== system TV_lisb/Subsystem/Tire Model/NaN handling1/Subsystem2 ==
  In1 : Inport
  If : If  IfExpression=u1 == 0
  If Action Subsystem : Subsystem  TreatAsAtomicUnit=on
  If Action Subsystem1 : Subsystem  TreatAsAtomicUnit=on
  Merge : Merge
  Relational Operator : RelationalOperator  Operator=isNaN  OutDataTypeStr=boolean  RndMeth=Simplest  InputSameDT=off
  Out1 : Outport
  wires:
  If Action Subsystem1/1(Out1) -> Merge/2
  In1/1 -> If Action Subsystem/1(In1), Relational Operator/1
  Merge/1 -> Out1/1
  If/2 -> If Action Subsystem1/Action
  If/1 -> If Action Subsystem/Action
  If Action Subsystem/1(Out1) -> Merge/1
  Relational Operator/1 -> If/1

== system TV_lisb/Subsystem/Tire Model/NaN handling1/Subsystem3 ==
  In1 : Inport
  If : If  IfExpression=u1 == 0
  If Action Subsystem : Subsystem  TreatAsAtomicUnit=on
  If Action Subsystem1 : Subsystem  TreatAsAtomicUnit=on
  Merge : Merge
  Relational Operator : RelationalOperator  Operator=isNaN  OutDataTypeStr=boolean  RndMeth=Simplest  InputSameDT=off
  Out1 : Outport
  wires:
  If Action Subsystem1/1(Out1) -> Merge/2
  In1/1 -> If Action Subsystem/1(In1), Relational Operator/1
  Merge/1 -> Out1/1
  If/2 -> If Action Subsystem1/Action
  If/1 -> If Action Subsystem/Action
  If Action Subsystem/1(Out1) -> Merge/1
  Relational Operator/1 -> If/1

== system TV_lisb/Subsystem/Vertical Loads/F-z calcs/Term_1 ==
  lr : Inport
  Acceleration_x : Inport  Port=2
  lf : Inport  Port=3
  hCG : Inport  Port=4
  g : Inport  Port=5
  Add : Sum
  Add1 : Sum
  Add2 : Sum  Inputs=+-
  Divide : Product  Inputs=*/
  Divide1 : Product  Inputs=**/
  Product : Product
  plus : Outport
  minus : Outport  Port=2
  wires:
  lr/1 -> Add/1, Divide/1
  lf/1 -> Add/2
  Add/1 -> Divide1/3, Divide/2
  Divide/1 -> Product/1
  g/1 -> Product/2
  Product/1 -> Add2/1, Add1/1
  hCG/1 -> Divide1/1
  Acceleration_x/1 -> Divide1/2
  Divide1/1 -> Add2/2, Add1/2
  Add1/1 -> plus/1
  Add2/1 -> minus/1
